simulink model "init_reset_val"  (R2019a)
settings: Solver=FixedStepDiscrete  StartTime=0.0  StopTime=100  FixedStep=1  RelTol=1e-3  SampleTimeConstraint=STIndependent
undefined symbols (not defined in the file): DiscIntNeverNeededParam
settings Model: Creator=The MathWorks, Inc.  LastModifiedBy=I22842
settings DataIOCC: SaveOutput=off  SaveTime=off
settings DebuggingCC: PregeneratedLibrarySubsystemCodeDiagnostic=none  ArithmeticOperatorsInVariantConditions=warning
settings SFSimCC: SimUseLocalCustomCode=off
settings RTWCC: GenCodeOnly=on  GenerateReport=on  RTWUseLocalCustomCode=off  LaunchReport=on
settings CodeAppCC: StateflowObjectComments=on
settings GRTTargetCC: MatFileLogging=off  SupportNonFinite=off
settings ConfigComp: CovMetricSettings=dswe

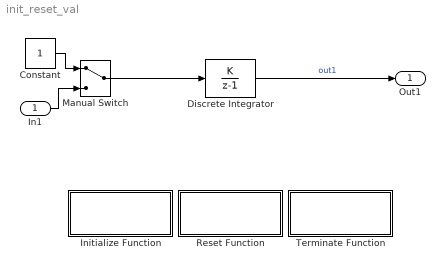
== system init_reset_val ==
  In1 : Inport
  Constant : Constant
  Discrete Integrator : DiscreteIntegrator  IntegratorMethod=Accumulation: Forward Euler  gainval=1  SampleTime=-1  ICPrevOutput=DiscIntNeverNeededParam  ICPrevScaledInput=DiscIntNeverNeededParam
  Initialize Function : Subsystem  TreatAsAtomicUnit=on
  Manual Switch : ManualSwitch
  Reset Function : Subsystem  TreatAsAtomicUnit=on
  Terminate Function : Subsystem  TreatAsAtomicUnit=on
  Out1 : Outport
  wires:
  Manual Switch/1 -> Discrete Integrator/1
  Discrete Integrator/1 -> Out1/1  "out1"
  Constant/1 -> Manual Switch/1
  In1/1 -> Manual Switch/2

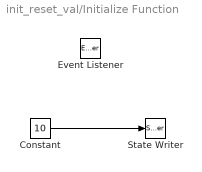
== system init_reset_val/Initialize Function ==
  Constant : Constant  DisableCoverage=on  Value=10
  Event Listener : EventListener  DisableCoverage=on  EventName=reset
  State Writer : StateWriter  DisableCoverage=on  StateOwnerBlock=../../Discrete Integrator
  wires:
  Constant/1 -> State Writer/1

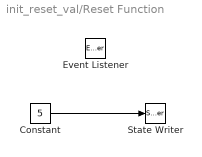
== system init_reset_val/Reset Function ==
  Constant : Constant  DisableCoverage=on  Value=5
  Event Listener : EventListener  DisableCoverage=on  EventType=Reset  EventName=reset
  State Writer : StateWriter  DisableCoverage=on  StateOwnerBlock=../../Discrete Integrator
  wires:
  Constant/1 -> State Writer/1

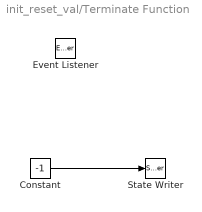
== system init_reset_val/Terminate Function ==
  Constant : Constant  DisableCoverage=on  Value=-1
  Event Listener : EventListener  DisableCoverage=on  EventType=Terminate  EventName=reset
  State Writer : StateWriter  DisableCoverage=on  StateOwnerBlock=../../Discrete Integrator
  wires:
  Constant/1 -> State Writer/1
